simulink model "AC_grid_Dynamic"  (R2025a)
settings: Solver=VariableStepAuto  StartTime=0.0  StopTime=10.0  RelTol=1e-3
undefined symbols (not defined in the file): C_Lines, Cbuses, fref, From_buses, From_nodes, L_Loads, Lines_fromM, Lines_toM, Load_buses, Nbuses, R_Lines, R_Loads, shift_lines, tap_lines, To_buses, To_nodes
(part 2 of 2)

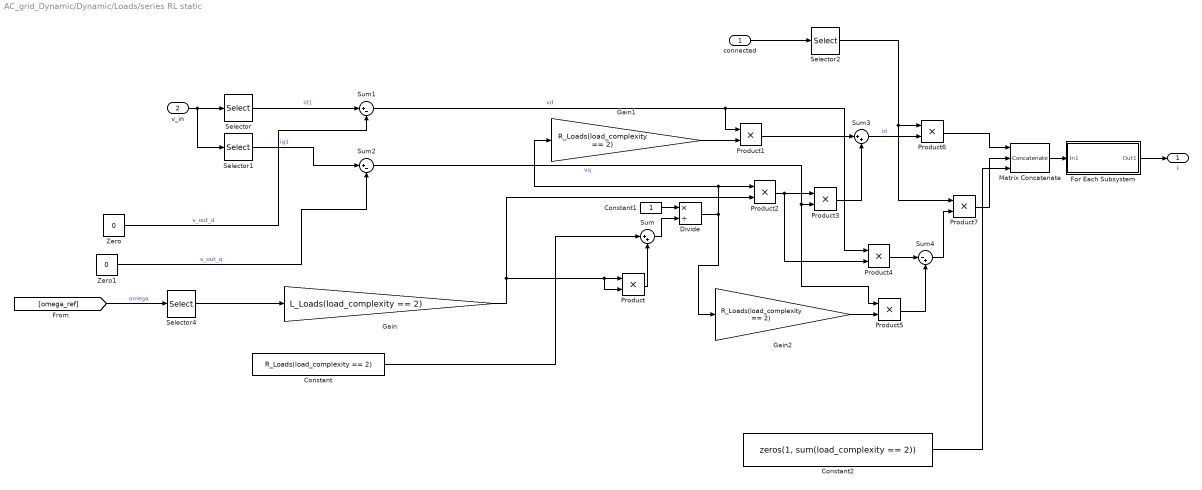
== system AC_grid_Dynamic/Dynamic/Loads/series RL static ==
  connected : Inport
  v_in : Inport  Port=2
  Constant : Constant  Value=R_Loads(load_complexity == 2)  VectorParams1D=off
  Constant1 : Constant
  Constant2 : Constant  Value=zeros(1, sum(load_complexity == 2))  VectorParams1D=off
  Divide : Product  Inputs=*/
  For Each Subsystem : Subsystem  TreatAsAtomicUnit=on
  Gain : Gain  Gain=L_Loads(load_complexity == 2)
  Gain1 : Gain  Gain=R_Loads(load_complexity == 2)
  Gain2 : Gain  Gain=R_Loads(load_complexity == 2)
  Matrix Concatenate : Concatenate  NumInputs=3  Mode=Multidimensional array
  Product{,1..7} (8 alike) : Product
  Selector : Selector  NumberOfDimensions=2  InputPortWidth=3  IndexOptions=Index vector (dialog),Index vector (dialog)  Indices=1,find(load_complexity == 2)  OutputSizes=1,1
  Selector1 : Selector  NumberOfDimensions=2  InputPortWidth=3  IndexOptions=Index vector (dialog),Index vector (dialog)  Indices=2,find(load_complexity == 2)  OutputSizes=1,1
  Selector2 : Selector  InputPortWidth=length(R_Loads)  IndexOptions=Index vector (dialog)  Indices=find(load_complexity == 2)  OutputSizes=1
  Selector4 : Selector  InputPortWidth=length(fref.ref_units)  IndexOptions=Index vector (dialog)  Indices=fref.loads(load_complexity == 2)  OutputSizes=1
  Sum : Sum  Inputs=|++
  Sum1 : Sum  Inputs=|+-
  Sum2 : Sum  Inputs=|+-
  Sum3 : Sum  Inputs=|++
  Sum4 : Sum  Inputs=|-+
  Zero : Constant  Value=0  OutDataTypeStr=Inherit: Inherit via back propagation
  Zero1 : Constant  Value=0  OutDataTypeStr=Inherit: Inherit via back propagation
  i : Outport
  wires:
  Selector4/1 -> Gain/1
  Constant/1 -> Sum/1
  Constant2/1 -> Matrix Concatenate/3
  For Each Subsystem/1(Out1) -> i/1
  Selector2/1 -> Product7/1, Product6/1
  Product6/1 -> Matrix Concatenate/1
  Matrix Concatenate/1 -> For Each Subsystem/1(In1)
  Selector1/1 -> Sum2/1  "iq1"
  Selector/1 -> Sum1/1  "id1"
  Product7/1 -> Matrix Concatenate/2
  Sum4/1 -> Product7/2
  Sum3/1 -> Product6/2  "id"
  connected/1 -> Selector2/1
  [omega_ref] -> Selector4/1  "omega"
  Zero1/1 -> Sum2/2  "v_out_q"
  Gain1/1 -> Product1/2
  Product2/1 -> Product4/2, Product3/1
  Product4/1 -> Sum4/1
  Divide/1 -> Gain2/1, Gain1/1, Product2/1
  Sum1/1 -> Product1/1, Product4/1  "vd"
  Product3/1 -> Sum3/2
  Constant1/1 -> Divide/1
  Gain/1 -> Product/2, Product/1, Product2/2
  Sum2/1 -> Product5/1, Product3/2  "vq"
  Product5/1 -> Sum4/2
  Product1/1 -> Sum3/1
  Product/1 -> Sum/2
  Gain2/1 -> Product5/2
  Sum/1 -> Divide/2
  Zero/1 -> Sum1/2  "v_out_d"
  v_in/1 -> Selector/1, Selector1/1

== system AC_grid_Dynamic/Dynamic/Loads/series RL static omega ==
  v_in : Inport
  connected : Inport  Port=2
  Constant1 : Constant  Value=zeros(1, sum(load_complexity == 3))  VectorParams1D=off
  For Each Subsystem : Subsystem  TreatAsAtomicUnit=on
  Gain : Gain  Gain=1./(R_Loads(load_complexity == 3).^2+L_Loads(load_complexity == 3).^2)
  Gain2 : Gain  Gain=1./(R_Loads(load_complexity == 3).^2+L_Loads(load_complexity == 3).^2)
  Gain3 : Gain  Gain=R_Loads(load_complexity == 3)
  Gain4 : Gain  Gain=L_Loads(load_complexity == 3)
  Gain5 : Gain  Gain=L_Loads(load_complexity == 3)
  Gain6 : Gain  Gain=R_Loads(load_complexity == 3)
  Matrix Concatenate : Concatenate  NumInputs=3  Mode=Multidimensional array
  Product2 : Product
  Product3 : Product
  Selector : Selector  NumberOfDimensions=2  InputPortWidth=3  IndexOptions=Index vector (dialog),Index vector (dialog)  Indices=1,find(load_complexity == 3)  OutputSizes=1,1
  Selector1 : Selector  NumberOfDimensions=2  InputPortWidth=3  IndexOptions=Index vector (dialog),Index vector (dialog)  Indices=2,find(load_complexity == 3)  OutputSizes=1,1
  Selector2 : Selector  InputPortWidth=length(R_Loads)  IndexOptions=Index vector (dialog)  Indices=find(load_complexity == 3)  OutputSizes=1
  Sum : Sum  Inputs=|++
  Sum3 : Sum  Inputs=|-+
  i : Outport
  wires:
  Constant1/1 -> Matrix Concatenate/3
  For Each Subsystem/1(Out1) -> i/1
  Selector2/1 -> Product3/1, Product2/1
  Product2/1 -> Matrix Concatenate/1
  Product3/1 -> Matrix Concatenate/2
  Matrix Concatenate/1 -> For Each Subsystem/1(In1)
  Selector1/1 -> Gain2/1  "iq1"
  Selector/1 -> Gain/1  "id1"
  Sum3/1 -> Product3/2
  Sum/1 -> Product2/2  "id"
  connected/1 -> Selector2/1
  v_in/1 -> Selector/1, Selector1/1
  Gain/1 -> Gain5/1, Gain3/1
  Gain3/1 -> Sum/1
  Gain4/1 -> Sum/2
  Gain2/1 -> Gain6/1, Gain4/1
  Gain5/1 -> Sum3/1
  Gain6/1 -> Sum3/2

== system AC_grid_Dynamic/Dynamic/Loads to buses/LoadsM ==
  i : Inport  Partition=on  PartitionDimension=1  PartitionWidth=1  PartitionOffset=0
  Assignment : Assignment  DiagnosticForDimensions=Warning  IndexOptions=Index vector (dialog)  Indices=Load_buses  OutputSizes=1
  For Each : ForEach  DisableCoverage=on
  Zero : Constant  Value=zeros(1,Nbuses)  VectorParams1D=off  OutDataTypeStr=Inherit: Inherit via back propagation
  Out1 : Outport  ConcatenationDimension=1
  wires:
  Zero/1 -> Assignment/1
  i/1 -> Assignment/2
  Assignment/1 -> Out1/1

== system AC_grid_Dynamic/Dynamic/iCbuses/Subsystem ==
  In1 : Inport
  State-Space : StateSpace  A=[]  B=[]  C=[]  D=Lines_toM  InitialCondition=0  ParameterTunability=Optimized
  State-Space1 : StateSpace  A=[]  B=[]  C=[]  D=Lines_fromM  InitialCondition=0  ParameterTunability=Optimized
  Sum : Sum  Inputs=|++
  Transpose : Math  Operator=transpose
  Transpose1 : Math  Operator=transpose
  Transpose2 : Math  Operator=transpose
  Out1 : Outport
  wires:
  In1/1 -> Transpose/1
  Transpose2/1 -> Sum/2
  Sum/1 -> Out1/1
  Transpose/1 -> State-Space/1, State-Space1/1
  State-Space/1 -> Transpose1/1
  State-Space1/1 -> Transpose2/1
  Transpose1/1 -> Sum/1

== system AC_grid_Dynamic/Dynamic/Buses/dynamic/For Each Subsystem ==
  In1 : Inport  Partition=on  PartitionDimension=1  PartitionWidth=1  PartitionOffset=0
  Assignment : Assignment  DiagnosticForDimensions=Warning  IndexOptions=Index vector (dialog)  Indices=find(bus_complexity == 1)  OutputSizes=1
  For Each : ForEach  DisableCoverage=on
  Zero : Constant  Value=zeros(1,Nbuses)  VectorParams1D=off  OutDataTypeStr=Inherit: Inherit via back propagation
  Out1 : Outport  ConcatenationDimension=1
  wires:
  Zero/1 -> Assignment/1
  Assignment/1 -> Out1/1
  In1/1 -> Assignment/2

== system AC_grid_Dynamic/Dynamic/Buses/only R/For Each Subsystem ==
  In1 : Inport  Partition=on  PartitionDimension=1  PartitionWidth=1  PartitionOffset=0
  Assignment : Assignment  DiagnosticForDimensions=Warning  IndexOptions=Index vector (dialog)  Indices=find(bus_complexity == 4)  OutputSizes=1
  For Each : ForEach  DisableCoverage=on
  Zero : Constant  Value=zeros(1,Nbuses)  VectorParams1D=off  OutDataTypeStr=Inherit: Inherit via back propagation
  Out1 : Outport  ConcatenationDimension=1
  wires:
  Zero/1 -> Assignment/1
  Assignment/1 -> Out1/1
  In1/1 -> Assignment/2

== system AC_grid_Dynamic/Dynamic/Buses/static/For Each Subsystem ==
  In1 : Inport  Partition=on  PartitionDimension=1  PartitionWidth=1  PartitionOffset=0
  Assignment : Assignment  DiagnosticForDimensions=Warning  IndexOptions=Index vector (dialog)  Indices=find(bus_complexity == 2)  OutputSizes=1
  For Each : ForEach  DisableCoverage=on
  Zero : Constant  Value=zeros(1,Nbuses)  VectorParams1D=off  OutDataTypeStr=Inherit: Inherit via back propagation
  Out1 : Outport  ConcatenationDimension=1
  wires:
  Zero/1 -> Assignment/1
  Assignment/1 -> Out1/1
  In1/1 -> Assignment/2

== system AC_grid_Dynamic/Dynamic/Buses/static omega/For Each Subsystem ==
  In1 : Inport  Partition=on  PartitionDimension=1  PartitionWidth=1  PartitionOffset=0
  Assignment : Assignment  DiagnosticForDimensions=Warning  IndexOptions=Index vector (dialog)  Indices=find(bus_complexity == 3)  OutputSizes=1
  For Each : ForEach  DisableCoverage=on
  Zero : Constant  Value=zeros(1,Nbuses)  VectorParams1D=off  OutDataTypeStr=Inherit: Inherit via back propagation
  Out1 : Outport  ConcatenationDimension=1
  wires:
  Zero/1 -> Assignment/1
  Assignment/1 -> Out1/1
  In1/1 -> Assignment/2

== system AC_grid_Dynamic/Dynamic/Buses/static omega/LPF ==
  in : Inport
  Gain : Gain  Gain=1e6
  I : Integrator  InitialCondition=[Grid_lf_op.op_report.Outputs(7).y(bus_complexity == 3); Grid_lf_op.op_report.Outputs(8).y(bus_complexity == 3); 0*Grid_lf_op.op_report.Outputs(7).y(bus_complexity == 3)]
  Sum4 : Sum  Inputs=|+-
  out : Outport
  wires:
  I/1 -> out/1, Sum4/2
  in/1 -> Sum4/1
  Sum4/1 -> Gain/1
  Gain/1 -> I/1

== system AC_grid_Dynamic/Dynamic/Lines/dynamic/For Each Subsystem ==
  In1 : Inport  Partition=on  PartitionDimension=1  PartitionWidth=1  PartitionOffset=0
  Assignment : Assignment  DiagnosticForDimensions=Warning  IndexOptions=Index vector (dialog)  Indices=find(line_complexity == 1)  OutputSizes=1
  For Each : ForEach  DisableCoverage=on
  Zero : Constant  Value=zeros(1,length(From_buses))  VectorParams1D=off  OutDataTypeStr=Inherit: Inherit via back propagation
  Out1 : Outport  ConcatenationDimension=1
  wires:
  Zero/1 -> Assignment/1
  Assignment/1 -> Out1/1
  In1/1 -> Assignment/2

== system AC_grid_Dynamic/Dynamic/Lines/static/For Each Subsystem ==
  In1 : Inport  Partition=on  PartitionDimension=1  PartitionWidth=1  PartitionOffset=0
  Assignment : Assignment  DiagnosticForDimensions=Warning  IndexOptions=Index vector (dialog)  Indices=find(line_complexity == 2)  OutputSizes=1
  For Each : ForEach  DisableCoverage=on
  Zero : Constant  Value=zeros(1,length(From_buses))  VectorParams1D=off  OutDataTypeStr=Inherit: Inherit via back propagation
  Out1 : Outport  ConcatenationDimension=1
  wires:
  Zero/1 -> Assignment/1
  Assignment/1 -> Out1/1
  In1/1 -> Assignment/2

== system AC_grid_Dynamic/Dynamic/Lines/static omega/For Each Subsystem ==
  In1 : Inport  Partition=on  PartitionDimension=1  PartitionWidth=1  PartitionOffset=0
  Assignment : Assignment  DiagnosticForDimensions=Warning  IndexOptions=Index vector (dialog)  Indices=find(line_complexity == 3)  OutputSizes=1
  For Each : ForEach  DisableCoverage=on
  Zero : Constant  Value=zeros(1,length(From_buses))  VectorParams1D=off  OutDataTypeStr=Inherit: Inherit via back propagation
  Out1 : Outport  ConcatenationDimension=1
  wires:
  Zero/1 -> Assignment/1
  Assignment/1 -> Out1/1
  In1/1 -> Assignment/2

== system AC_grid_Dynamic/Dynamic/Loads/PQ/For Each Subsystem ==
  In1 : Inport  Partition=on  PartitionDimension=1  PartitionWidth=1  PartitionOffset=0
  Assignment : Assignment  DiagnosticForDimensions=Warning  IndexOptions=Index vector (dialog)  Indices=find(load_complexity == 4)  OutputSizes=1
  For Each : ForEach  DisableCoverage=on
  Zero : Constant  Value=zeros(1,length(L_Loads))  VectorParams1D=off  OutDataTypeStr=Inherit: Inherit via back propagation
  Out1 : Outport  ConcatenationDimension=1
  wires:
  Zero/1 -> Assignment/1
  Assignment/1 -> Out1/1
  In1/1 -> Assignment/2

== system AC_grid_Dynamic/Dynamic/Loads/dynamic PQ/For Each Subsystem ==
  In1 : Inport  Partition=on  PartitionDimension=1  PartitionWidth=1  PartitionOffset=0
  Assignment : Assignment  DiagnosticForDimensions=Warning  IndexOptions=Index vector (dialog)  Indices=find(load_complexity == 5)  OutputSizes=1
  For Each : ForEach  DisableCoverage=on
  Zero : Constant  Value=zeros(1,length(L_Loads))  VectorParams1D=off  OutDataTypeStr=Inherit: Inherit via back propagation
  Out1 : Outport  ConcatenationDimension=1
  wires:
  Zero/1 -> Assignment/1
  Assignment/1 -> Out1/1
  In1/1 -> Assignment/2

== system AC_grid_Dynamic/Dynamic/Loads/dynamic PQ/i_d ==
  in : Inport
  Gain : Gain  Gain=1./T_s
  I : Integrator  InitialCondition=Grid_lf_op.op_report.Outputs(5).y(load_complexity == 5)
  Sum4 : Sum  Inputs=|+-
  out : Outport
  wires:
  I/1 -> Sum4/2, out/1
  in/1 -> Sum4/1
  Sum4/1 -> Gain/1
  Gain/1 -> I/1

== system AC_grid_Dynamic/Dynamic/Loads/dynamic PQ/i_q ==
  in : Inport
  Gain : Gain  Gain=1./T_s
  I : Integrator  InitialCondition=Grid_lf_op.op_report.Outputs(6).y(load_complexity == 5)
  Sum4 : Sum  Inputs=|+-
  out : Outport
  wires:
  Gain/1 -> I/1
  Sum4/1 -> Gain/1
  in/1 -> Sum4/1
  I/1 -> out/1, Sum4/2

== system AC_grid_Dynamic/Dynamic/Loads/parallel RL dynamic/For Each Subsystem ==
  In1 : Inport  Partition=on  PartitionDimension=1  PartitionWidth=1  PartitionOffset=0
  Assignment : Assignment  DiagnosticForDimensions=Warning  IndexOptions=Index vector (dialog)  Indices=find(load_complexity == 6)  OutputSizes=1
  For Each : ForEach  DisableCoverage=on
  Zero : Constant  Value=zeros(1,length(L_Loads))  VectorParams1D=off  OutDataTypeStr=Inherit: Inherit via back propagation
  Out1 : Outport  ConcatenationDimension=1
  wires:
  In1/1 -> Assignment/2
  Assignment/1 -> Out1/1
  Zero/1 -> Assignment/1

== system AC_grid_Dynamic/Dynamic/Loads/parallel RL static/For Each Subsystem ==
  In1 : Inport  Partition=on  PartitionDimension=1  PartitionWidth=1  PartitionOffset=0
  Assignment : Assignment  DiagnosticForDimensions=Warning  IndexOptions=Index vector (dialog)  Indices=find(load_complexity == 1)  OutputSizes=1
  For Each : ForEach  DisableCoverage=on
  Zero : Constant  Value=zeros(1,length(L_Loads))  VectorParams1D=off  OutDataTypeStr=Inherit: Inherit via back propagation
  Out1 : Outport  ConcatenationDimension=1
  wires:
  Zero/1 -> Assignment/1
  Assignment/1 -> Out1/1
  In1/1 -> Assignment/2

== system AC_grid_Dynamic/Dynamic/Loads/parallel RL static omega/For Each Subsystem ==
  In1 : Inport  Partition=on  PartitionDimension=1  PartitionWidth=1  PartitionOffset=0
  Assignment : Assignment  DiagnosticForDimensions=Warning  IndexOptions=Index vector (dialog)  Indices=find(load_complexity == 1)  OutputSizes=1
  For Each : ForEach  DisableCoverage=on
  Zero : Constant  Value=zeros(1,length(L_Loads))  VectorParams1D=off  OutDataTypeStr=Inherit: Inherit via back propagation
  Out1 : Outport  ConcatenationDimension=1
  wires:
  In1/1 -> Assignment/2
  Assignment/1 -> Out1/1
  Zero/1 -> Assignment/1

== system AC_grid_Dynamic/Dynamic/Loads/series RL dynamic/For Each Subsystem ==
  In1 : Inport  Partition=on  PartitionDimension=1  PartitionWidth=1  PartitionOffset=0
  Assignment : Assignment  DiagnosticForDimensions=Warning  IndexOptions=Index vector (dialog)  Indices=find(load_complexity == 1)  OutputSizes=1
  For Each : ForEach  DisableCoverage=on
  Zero : Constant  Value=zeros(1,length(L_Loads))  VectorParams1D=off  OutDataTypeStr=Inherit: Inherit via back propagation
  Out1 : Outport  ConcatenationDimension=1
  wires:
  Zero/1 -> Assignment/1
  Assignment/1 -> Out1/1
  In1/1 -> Assignment/2

== system AC_grid_Dynamic/Dynamic/Loads/series RL static/For Each Subsystem ==
  In1 : Inport  Partition=on  PartitionDimension=1  PartitionWidth=1  PartitionOffset=0
  Assignment : Assignment  DiagnosticForDimensions=Warning  IndexOptions=Index vector (dialog)  Indices=find(load_complexity == 2)  OutputSizes=1
  For Each : ForEach  DisableCoverage=on
  Zero : Constant  Value=zeros(1,length(L_Loads))  VectorParams1D=off  OutDataTypeStr=Inherit: Inherit via back propagation
  Out1 : Outport  ConcatenationDimension=1
  wires:
  Zero/1 -> Assignment/1
  Assignment/1 -> Out1/1
  In1/1 -> Assignment/2

== system AC_grid_Dynamic/Dynamic/Loads/series RL static omega/For Each Subsystem ==
  In1 : Inport  Partition=on  PartitionDimension=1  PartitionWidth=1  PartitionOffset=0
  Assignment : Assignment  DiagnosticForDimensions=Warning  IndexOptions=Index vector (dialog)  Indices=find(load_complexity == 3)  OutputSizes=1
  For Each : ForEach  DisableCoverage=on
  Zero : Constant  Value=zeros(1,length(L_Loads))  VectorParams1D=off  OutDataTypeStr=Inherit: Inherit via back propagation
  Out1 : Outport  ConcatenationDimension=1
  wires:
  Zero/1 -> Assignment/1
  Assignment/1 -> Out1/1
  In1/1 -> Assignment/2
